simulink model "TricycleBotControl"  (R2021a)
settings: Solver=ode45  StartTime=0.0  StopTime=20  RelTol=1e-3  EnableMultiTasking=on
values from neighbouring files (symbols this model uses):
  Tstep = 0.01    [PurePursuitMain.m]
  x0 = 1    [PurePursuitMain.m]
libraries: simulink x1
settings Model: Creator=Gu  LastModifiedBy=duong
settings SolverCC: AlgebraicLoopSolver=TrustRegion
settings DataIOCC: LimitDataPoints=on  SaveFormat=Array  SignalLoggingSaveFormat=ModelDataLogs  ReturnWorkspaceOutputs=off
settings OptimizationCC: ExpressionDepthLimit=2147483647  LifeSpan=inf
settings DebuggingCC: UnderspecifiedInitializationDetection=Classic  MergeDetectMultiDrivingBlocksExec=none  FcnCallInpInsideContextMsg=warning  StateNameClashWarn=warning  SFUnexpectedBacktrackingDiag=warning  SFNoUnconditionalDefaultTransitionDiag=warning  SFMachineParentedDataDiag=warning  ArithmeticOperatorsInVariantConditions=warning
settings HardwareCC: ProdBitPerPointer=32  ProdBitPerSizeT=32  ProdBitPerPtrDiffT=32  ProdLargestAtomicFloat=None  ProdIntDivRoundTo=Undefined  ProdEndianess=Unspecified  ProdWordSize=32  ProdHWDeviceType=32-bit Generic
settings ModelReferenceCC: PropagateSignalLabelsOutOfModel=off
settings SFSimCC: SimUseLocalCustomCode=off  SimParseCustomCode=off  CustomCodeUndefinedFunction=UseInterfaceOnly
settings RTWCC: RTWUseLocalCustomCode=off
settings CodeAppCC: StateflowObjectComments=on
settings GRTTargetCC: TargetLangStandard=C89/C90 (ANSI)  CombineOutputUpdateFcns=off  GRTInterface=on
settings ConfigComp: CovMetricSettings=dw  CovSaveCumulativeToWorkspaceVar=on  CovSaveSingleToWorkspaceVar=on  CovExternalEMLEnable=off  CovSFcnEnable=off

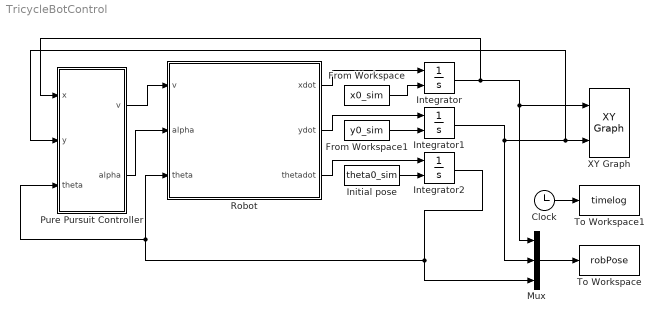
== system TricycleBotControl ==
  Clock : Clock
  From Workspace : FromWorkspace  VariableName=x0_sim  OutputAfterFinalValue=Holding final value
  From Workspace1 : FromWorkspace  VariableName=y0_sim  OutputAfterFinalValue=Holding final value
  Initial pose : FromWorkspace  VariableName=theta0_sim  OutputAfterFinalValue=Holding final value
  Integrator : Integrator  InitialConditionSource=external  InitialCondition=x0
  Integrator1 : Integrator  InitialConditionSource=external  InitialCondition=2
  Integrator2 : Integrator  InitialConditionSource=external  InitialCondition=pi/4
  Mux : Mux  Inputs=3
  Pure Pursuit Controller : MATLAB Function  TreatAsAtomicUnit=on
  Robot : MATLAB Function  TreatAsAtomicUnit=on
  To Workspace : ToWorkspace  VariableName=robPose  SampleTime=Tstep
  To Workspace1 : ToWorkspace  VariableName=timelog  SampleTime=-1
      settings: Save2DSignal=2-D array (concatenate along first dimension)
  XY Graph : simulink/Sinks/XY Graph  xmin=-10  xmax=10  ymin=-10  ymax=10  st=-1
  wires:
  Robot/1(xdot) -> Integrator/1
  Robot/2(ydot) -> Integrator1/1
  Robot/3(thetadot) -> Integrator2/1
  Integrator2/1 -> Robot/3(theta), Pure Pursuit Controller/3(theta), Mux/3
  Integrator/1 -> Pure Pursuit Controller/1(x), XY Graph/1, Mux/1
  Integrator1/1 -> Pure Pursuit Controller/2(y), XY Graph/2, Mux/2
  Clock/1 -> To Workspace1/1
  Pure Pursuit Controller/1(v) -> Robot/1(v)
  Pure Pursuit Controller/2(alpha) -> Robot/2(alpha)
  Mux/1 -> To Workspace/1
  From Workspace/1 -> Integrator/2
  From Workspace1/1 -> Integrator1/2
  Initial pose/1 -> Integrator2/2

== matlab function TricycleBotControl/Pure Pursuit Controller ==
  data: v output; alpha output; x input; y input; theta input
% This implementation assumes that the robot moves along waypoints 
% with increasing x coordinates
function [v,alpha] = fcn(x,y,theta)

% Look ahead distance:
L = 0.3;

wp=[1,2;5,2;5.8,1.55;7.95,1;10.95 1];
xint=zeros(1);
yint=zeros(1);

for i=1:numrows(wp)-1
    wpNum = ceil(abs(wp(i+1)-wp(i))/(0.1*L));
    xt =zeros(wpNum,1);
    for j=1:wpNum
        xt(j,1)=wp(i,1)+(j-1)*(0.1*L);
    end
    yt=interp1(wp(i:i+1,1),wp(i:i+1,2),xt);
    xint=[xint;xt];
    yint=[yint;yt];
end

% Find the next waypoint
goal = [x,y];
for i=1:length(xint)
    if x < xint(i) && norm([xint(i) yint(i)]-[x,y])>= L
        goal = [xint(i) yint(i)];
        break;
    elseif x < xint(i)
        goal = [xint(i) yint(i)];
        break;        
    end
end

if isequal(goal,[x,y])
    alpha = 0;
    v = 0; % Constant velocity
else
    v = 0.5; % Constant velocity
    % Calculate the turning angle
    if abs(goal(2)-y) == 0
        alpha = 0;
    else
        % Ref: https://vinesmsuic.github.io/2020/09/29/robotics-purepersuit/#curvature-of-arc
        a = -tan(theta);
        b = 1;
        c = tan(theta)*x-y;
        Distance = abs(a*goal(1)+b*goal(2)+c)/norm([a b]);

        side = -sign(sin(theta)*(goal(1)-x) - cos(theta)*(goal(2)-y));
        alpha = side*L^2/(2*Distance);
    end
end

== matlab function TricycleBotControl/Robot ==
  data: v input; xdot output; alpha input; theta input; ydot output; thetadot output
function [xdot, ydot, thetadot] = fcn(v, alpha, theta)

d = 1;  % axial space

% Kinematic equations
xdot=v*cos(theta);
ydot=v*sin(theta);
thetadot=v*tan(alpha)/d;
